simulink model "sim_2D_paper_recreation"  (R2024b)
settings: Solver=FixedStepAuto  StartTime=0.0  StopTime=300  FixedStep=0.0001  RelTol=1e-3
settings Model: Creator=olive  LastModifiedBy=olive
settings DebuggingCC: UnderSpecifiedDimensionMsg=warning

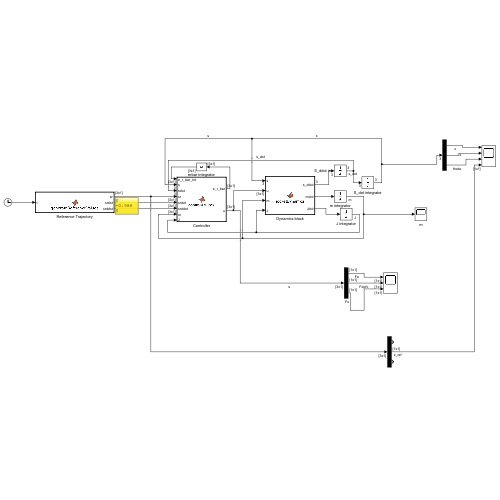
[thumbnail: Simulink's stored preview of the top-level diagram]
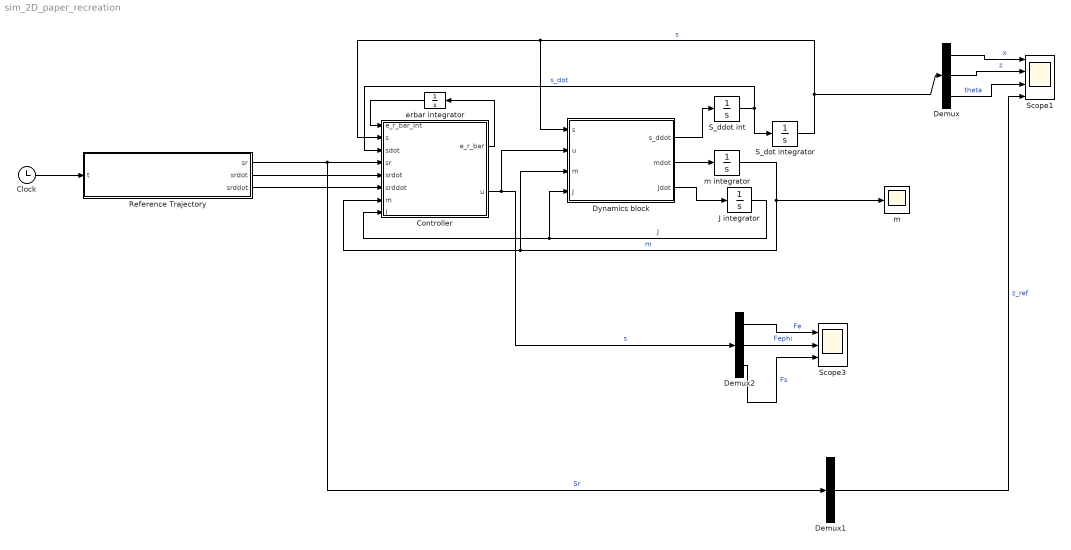
== system sim_2D_paper_recreation ==
  Clock : Clock
  Controller : MATLAB Function  TreatAsAtomicUnit=on
  Demux : Demux  Outputs=3
  Demux1 : Demux  Outputs=3
  Demux2 : Demux  Outputs=3
  Dynamics block : MATLAB Function  TreatAsAtomicUnit=on
  J integrator : Integrator  InitialCondition=5
  Reference Trajectory : MATLAB Function  TreatAsAtomicUnit=on
  S_ddot int : Integrator  InitialCondition=[0; 0; 0]
  S_dot integrator : Integrator  InitialCondition=[0.3;1;0]
  Scope1 : Scope  NumInputPorts=4
  Scope3 : Scope  NumInputPorts=3
  erbar integrator : Integrator
  m : Scope
  m integrator : Integrator  InitialCondition=25
  wires:
  Dynamics block/1(s_ddot) -> S_ddot int/1
  Dynamics block/2(mdot) -> m integrator/1
  Dynamics block/3(Jdot) -> J integrator/1
  S_ddot int/1 -> S_dot integrator/1, Controller/3(sdot)  "s_dot"
  S_dot integrator/1 -> Dynamics block/1(s), Controller/2(s), Demux/1  "s"
  J integrator/1 -> Dynamics block/4(J), Controller/8(J)  "J"
  m integrator/1 -> Dynamics block/3(m), Controller/7(m), m/1  "m"
  Controller/1(e_r_bar) -> erbar integrator/1
  erbar integrator/1 -> Controller/1(e_r_bar_Int)
  Demux/1 -> Scope1/1  "x"
  Demux/2 -> Scope1/2  "z"
  Demux/3 -> Scope1/3  "theta"
  Demux2/2 -> Scope3/2  "Fephi"
  Demux2/1 -> Scope3/1  "Fe"
  Controller/2(u) -> Demux2/1, Dynamics block/2(u)  "s"
  Demux2/3 -> Scope3/3  "Fs"
  Clock/1 -> Reference Trajectory/1(t)
  Reference Trajectory/1(sr) -> Demux1/1, Controller/4(sr)  "Sr"
  Reference Trajectory/3(srddot) -> Controller/6(srddot)
  Reference Trajectory/2(srdot) -> Controller/5(srdot)
  Demux1/2 -> Scope1/4  "z_ref"

== matlab function sim_2D_paper_recreation/Reference Trajectory ==
  data: sr output; srdot output; srddot output; t input
function [sr, srdot, srddot] = generateReferenceValues(t)
% Generates constant reference position and velocity values for x, z, and theta
% Outputs:
%   sr: Reference position vector [x_ref; z_ref; theta_ref]
%   srdot: Reference velocity vector [x_dot_ref; z_dot_ref; theta_dot_ref]

%set position and time for each segment
%the rocket follows a trajectory of a half sine wave (middle part) then a
%semi circle for the top of the boostback portion 
%then a straight line downwards

    % Reference positions
    x_ref = 0;    % Reference x position (m)
    if t>20 && t<25
        z_ref = 0.016*t^3 - 1.08*t^2 +24*t -175;    %reference position 
    else 
        if t >25
            z_ref = 0; %set final value
        else
            z_ref = 1;
        end
    end
    theta_ref = 0; % Reference theta position (rad)

    % Reference velocities
    x_dot_ref = 0;    % Reference x velocity (m/s)
    if t>20 && t<25
        z_dot_ref = 0.048*t^2 - 2.16*t +24;    %reference position 
    else 
        z_dot_ref = 0; %set final value
    end
    % z_dot_ref = 0.1*cos(0.1*t);
    theta_dot_ref = 0; % Reference theta velocity (rad/s)

    % Reference accelerations
    x_ddot_ref = 0;    % Reference x velocity (m/s)
    if t>20 && t<25
        z_ddot_ref = 0.096*t - 2.16;    % Reference z position (m)
    else
        z_ddot_ref = 0;
    end
    % z_ddot_ref = -0.01*sin(0.1*t);
    theta_ddot_ref = 0; % Reference theta velocity (rad/s)

    % Output reference values
    sr = [x_ref; z_ref; theta_ref];
    srdot = [x_dot_ref; z_dot_ref; theta_dot_ref];
    srddot = [x_ddot_ref; z_ddot_ref; theta_ddot_ref];
end

== matlab function sim_2D_paper_recreation/Dynamics block ==
  data: s input size=3; u input; m input; J input; s_ddot output size=3; mdot output size=1; Jdot output size=1
function [s_ddot,mdot,Jdot] = rocketDynamics(s,u,m,J)

%initialise states
L1 = 1;
L2 = 1;
Ln = 1;
alpha1 = 0.009;
alpha2 = 0.005;
beta = 0.03;
g = 9.81;

%extract states
Fe = u(1);
Fephi = u(2);
Fs = u(3);
theta = s(3);

%find mdot and Jdot
mdot = -alpha1*(beta*Fe +abs(Fs));
Jdot = -alpha2*(beta*Fe + abs(Fs));
%update mdot and Jdot

fs = [0;-g;0];
gs = [theta/m 1/m 1/m; 1/m -theta/m -theta/m; 0 -(L1+Ln)/J L2/J]; 
s_ddot = fs + gs * u;
end

== matlab function sim_2D_paper_recreation/Controller ==
  data: e_r_bar_Int input; s input; sdot input; sr input; srdot input; srddot input; m input; J input; e_r_bar output; u output
function [e_r_bar,u] = controllerBlock(e_r_bar_Int,s,sdot,sr,srdot,srddot,m,J)
% controllerBlock computes control input u for a 3-DOF system.
%
% Inputs:
%   s       = [x; z; theta] (actual position/orientation)
%   sr      = [x_r; z_r; theta_r] (reference)
%   sdot    = [xdot; zdot; thetadot] (actual velocity)
%   srdot   = [x_rdot; z_rdot; theta_rdot] (reference velocity)
%   sddot   = [xddot; zddot; thetaddot] (actual acceleration)
%   srddot  = [x_rddot; z_rddot; theta_rddot] (reference acceleration)
%
% Output:
%   u       = control input 

    % == Extract actual states ==
    x       = s(1); 
    z       = s(2);
    theta   = s(3);
    
    % == Extract reference states ==
    xr      = sr(1);
    zr      = sr(2);
    thetar  = sr(3);

    % == Extract actual velocities ==
    xdot    = sdot(1);
    zdot    = sdot(2);
    thetadot= sdot(3);

    % == Extract reference velocities ==
    xrdot   = srdot(1);
    zrdot   = srdot(2);
    thetardot = srdot(3);

    % == Constants / Gains (fill in correct values!) ==
    g       = 9.81;     % Gravity
    L1      = 1;      % etc... fill in or remove as needed
    L2      = 1;
    Ln      = 1;
    kx      = 5;        % Gains for position errors
    kz      = 6;
    ktheta  = 5;
    
    % define f_s
    f_s = [0; -g; 0];  
   
    % Define gs
    g_s = [ theta/m   1/m   1/m;
            1/m    -theta/m  -theta/m;
            0     -(L1+Ln)/J     L2/J ];
        
    % Gains for the error feedback
    K_s = diag([0.5, 0.1, 0.25]);
    K_i = diag([0.25, 0.0, 0.25]);  
    K_r = diag([kx, kz, ktheta]);   
    
    % == Errors ==
    % Position error:
    e_pos  = [x - xr; z - zr; theta - thetar];
    
    % Velocity error:
    e_vel  = [xdot - xrdot; zdot - zrdot; thetadot - thetardot];  

    % == Now compute your feedforward and feedback terms ==
    f_s_bar = f_s - srddot + K_r * e_vel; 
  

    e_r_bar = e_vel + K_r * e_pos;  

    % == Calculate u 
    u = g_s\( -f_s_bar - K_s * e_r_bar - K_i * e_r_bar_Int );
    
    %set bounds for u 
    u(1) =  max(0, min(6486, u(1)));  %We need to bound Fe min = 0N max = 6486N
    u(2) =  max(-1678.7, min(1678.7, u(2)));  %Need to Bound Fephi 
    u(3) =  max(-130, min(130, u(3)));  %Need to bound Fs

end
